simulink library "dspsnks2"  (Simulink 3.00)
undefined symbols (not defined in the file or in its folder): get, hot
libraries: dspspect2 x2, dspmtrx2 x2, dspbuff2 x1, dspsnks2 x1
settings Model: Creator=don  LastModifiedBy=don

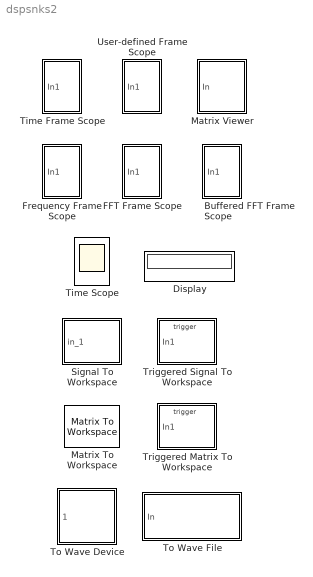
== system dspsnks2 ==
  Buffered FFT Frame Scope : Subsystem  mask(Buffered FFT Frame Scope){FFTlength=128, BufferSize=128, Overlap=64, Domain=Frequency, XLabel=Samples, XUnits=Hertz, XRange=[0...Fs/2], XIncr=-1, YLabel=Magnitude, dB, YUnits=dB, HorizSpan=1, NChans=1, AxisParams=off, YMin=-10, YMax=10, FigPos=get(0,'defaultfigureposition'), AxisGrid=on, AxisZoom=on, FrameNumber=off, AxisLegend=off, Memory=off, LineParams=off, LineDisables=, LineColors=, LineStyles=, LineMarkers=}
      mask prompts: FFTlength "FFT length (-1 to inherit input width):"; BufferSize "Buffer size:"; Overlap "Buffer overlap:"; Domain "Input domain:"; XLabel "X-axis title:"; XUnits "Frequency units:"; XRange "Frequency range:"; XIncr "Sample time of original time series (-1 if not zero-padded):"; YLabel "Y-axis title:"; YUnits "Amplitude scaling:"; HorizSpan "Time display span (number of frames):"; NChans "Number of input channels:"; AxisParams "Axis properties ..."; YMin "Minimum Y-limit:"; YMax "Maximum Y-limit:"; FigPos "Figure position:"; AxisGrid "Axis grid"; AxisZoom "Axis zoom"; FrameNumber "Frame number"; AxisLegend "Axis legend"; LineParams "Line properties ..."; LineDisables "Line visibility:"; LineColors "Line colors:"; LineStyles "Line styles:"; LineMarkers "Line markers:"
      mask help: Buffer a non-frame based input, then compute and display the magnitude-squared FFT of each each frame of input data.
      mask init:
      | [x,y,str] = dspblkbfftscope('icon');
      | s = dspblkbfftscope('init',FFTlength,BufferSize,Overlap,Domain, XLabel, XUnits, XRange, XIncr, ...
      | YLabel, YUnits,  HorizSpan, NChans, ...
      | AxisParams, YMin,YMax,FigPos, ...
      | AxisGrid, AxisZoom, FrameNumber, AxisLegend, Memory, ...
      | LineParams, LineDisables, LineColors, LineStyles, LineMarkers);
      settings: CopyFcn=sdspfscope([],[],[],'BlockCopy');  DeleteFcn=sdspfscope([],[],[],'BlockDelete');  NameChangeFcn=sdspfscope([],[],[],'NameChange');
      mask Help: web(dspbhelp);
      mask StyleString: edit,edit,edit,popup(Time|Frequency|User-defined),edit,popup(Hertz|rad/sec),popup([0...Fs/2]|[-Fs/2...Fs/2]|[0...Fs]),edit,edit,popup(Magnitude|dB),edit,edit,checkbox,edit,edit,edit,checkbox,checkbox,checkbox,checkbox,checkbox,checkbox,edit,edit,edit,edit
      mask CallbackString: |||dspblkbfftscope('dynamic','Domain');|||||||||dspblkbfftscope('dynamic','AxisParams');|||||||||dspblkbfftscope('dynamic','LineParams');||||
      mask Display: plot(x,y); text(14,20,str);
  Display : Display
      settings: Format=short
  FFT Frame Scope : Subsystem  mask(FFT Frame Scope){FFTlength=128, Domain=Frequency, XLabel=Samples, XUnits=Hertz, XRange=[0...Fs/2], XIncr=-1, YLabel=Magnitude, dB, YUnits=dB, HorizSpan=1, NChans=1, AxisParams=off, YMin=-10, YMax=10, FigPos=get(0,'defaultfigureposition'), AxisGrid=on, AxisZoom=on, FrameNumber=off, AxisLegend=off, Memory=off, LineParams=off, LineDisables=, LineColors=, LineStyles=, LineMarkers=}
      mask prompts: FFTlength "FFT length (-1 to inherit input width):"; Domain "Input domain:"; XLabel "X-axis title:"; XUnits "Frequency units:"; XRange "Frequency range:"; XIncr "Sample time of original time series (-1 if not zero-padded):"; YLabel "Y-axis title:"; YUnits "Amplitude scaling:"; HorizSpan "Time display span (number of frames):"; NChans "Number of input channels:"; AxisParams "Axis properties ..."; YMin "Minimum Y-limit:"; YMax "Maximum Y-limit:"; FigPos "Figure position:"; AxisGrid "Axis grid"; AxisZoom "Axis zoom"; FrameNumber "Frame number"; AxisLegend "Axis legend"; LineParams "Line properties ..."; LineDisables "Line visibilities:"; LineColors "Line colors:"; LineStyles "Line styles:"; LineMarkers "Line markers:"
      mask help: Compute and display the magnitude-squared FFT of a frame of time-domain input data.
      mask init:
      | [x,y,str] = dspblkfftscope('icon');
      | s = dspblkfftscope('init',FFTlength,Domain, XLabel, XUnits, XRange, XIncr, ...
      | YLabel, YUnits,  HorizSpan, NChans, ...
      | AxisParams, YMin,YMax,FigPos, ...
      | AxisGrid, AxisZoom, FrameNumber, AxisLegend, Memory, ...
      | LineParams, LineDisables, LineColors, LineStyles, LineMarkers);
      settings: CopyFcn=sdspfscope([],[],[],'BlockCopy');  DeleteFcn=sdspfscope([],[],[],'BlockDelete');  NameChangeFcn=sdspfscope([],[],[],'NameChange');
      mask Help: web(dspbhelp);
      mask StyleString: edit,popup(Time|Frequency|User-defined),edit,popup(Hertz|rad/sec),popup([0...Fs/2]|[-Fs/2...Fs/2]|[0...Fs]),edit,edit,popup(Magnitude|dB),edit,edit,checkbox,edit,edit,edit,checkbox,checkbox,checkbox,checkbox,checkbox,checkbox,edit,edit,edit,edit
      mask CallbackString: |dspblkfftscope('dynamic','Domain');|||||||||dspblkfftscope('dynamic','AxisParams');|||||||||dspblkfftscope('dynamic','LineParams');||||
      mask Display: plot(x,y); text(14,20,str);
  Frequency Frame Scope : Subsystem  mask(Frequency Frame Scope){Domain=Frequency, XLabel=Samples, XUnits=Hertz, XRange=[0...Fs/2], XIncr=-1, YLabel=Magnitude, dB, YUnits=dB, HorizSpan=1, NChans=1, AxisParams=off, YMin=-10, YMax=10, FigPos=get(0,'defaultfigureposition'), AxisGrid=on, AxisZoom=on, FrameNumber=off, AxisLegend=off, Memory=off, LineParams=off, LineDisables=, LineColors=, LineStyles=, LineMarkers=}
      mask prompts: Domain "Input domain:"; XLabel "X-axis title:"; XUnits "Frequency units:"; XRange "Frequency range:"; XIncr "Sample time of original time series (-1 if not zero-padded):"; YLabel "Y-axis title:"; YUnits "Amplitude scaling:"; HorizSpan "Time display span (number of frames):"; NChans "Number of input channels:"; AxisParams "Axis properties ..."; YMin "Minimum Y-limit:"; YMax "Maximum Y-limit:"; FigPos "Figure position:"; AxisGrid "Axis grid"; AxisZoom "Axis zoom"; FrameNumber "Frame number"; AxisLegend "Axis legend"; LineParams "Line properties ..."; LineDisables "Line visibilities:"; LineColors "Line colors:"; LineStyles "Line styles:"; LineMarkers "Line markers:"
      mask help: Display one or more frequency domain data sets. Data should come from an FFT block, or from frequency-domain sources with equivalent data organization.
      mask init:
      | [x,y,str] = dspblkfscope('icon');
      | s = dspblkfscope('init',Domain, XLabel, XUnits, XRange, XIncr, ...
      | YLabel, YUnits,  HorizSpan, NChans, ...
      | AxisParams, YMin,YMax,FigPos, ...
      | AxisGrid, AxisZoom, FrameNumber, AxisLegend, Memory, ...
      | LineParams, LineDisables, LineColors, LineStyles, LineMarkers);
      settings: CopyFcn=sdspfscope([],[],[],'BlockCopy');  DeleteFcn=sdspfscope([],[],[],'BlockDelete');  NameChangeFcn=sdspfscope([],[],[],'NameChange');
      mask Help: web(dspbhelp);
      mask StyleString: popup(Time|Frequency|User-defined),edit,popup(Hertz|rad/sec),popup([0...Fs/2]|[-Fs/2...Fs/2]|[0...Fs]),edit,edit,popup(Magnitude|dB),edit,edit,checkbox,edit,edit,edit,checkbox,checkbox,checkbox,checkbox,checkbox,checkbox,edit,edit,edit,edit
      mask CallbackString: dspblkfscope('dynamic','Domain');|||||||||dspblkfscope('dynamic','AxisParams');|||||||||dspblkfscope('dynamic','LineParams');||||
      mask Display: plot(x,y); text(14,20,str);
  Matrix To Workspace : dspmtrx2/Matrix To Workspace  matname=yout  maxrows=1000  deci=1  matsiz=[3 3]
  Matrix Viewer : Subsystem  mask(Matrix Viewer){ImageParams=off, CMap=hot(256), YMin=-1.0, YMax=1.0, NumCols=10, AxisColorbar=on, AxisParams=off, AxisOrigin=Upper left corner, XLabel=X-axis, YLabel=Y-axis, ZLabel=Z-axis, FigPos=get(0,'defaultfigureposition'), AxisZoom=off}
      mask prompts: ImageParams "Image properties ..."; CMap "Colormap matrix:"; YMin "Minimum input value:"; YMax "Maximum input value:"; NumCols "Number of columns:"; AxisColorbar "Display colorbar"; AxisParams "Axis properties ..."; AxisOrigin "Axis origin:"; XLabel "X-axis title:"; YLabel "Y-axis title:"; ZLabel "Colorbar title:"; FigPos "Figure position:"; AxisZoom "Axis zoom"
      mask help: Display a matrix as an image, scaling the colormap to the specified input data range. Colormap must be an Nx3 matrix of RGB values. Type "help graph3d" at the MATLAB prompt for a list of predefined colormaps.
      mask init:
      | s = dspblkmview('init', ...
      |        ImageParams, CMap, YMin, YMax, NumCols, AxisColorbar,  ...
      |        AxisParams,  AxisOrigin, XLabel,  YLabel,  ZLabel, FigPos, AxisZoom);
      settings: CopyFcn=sdspmview([],[],[],'BlockCopy');  DeleteFcn=sdspmview([],[],[],'BlockDelete');  NameChangeFcn=sdspmview([],[],[],'NameChange');
      mask Help: web(dspbhelp);
      mask StyleString: checkbox,edit,edit,edit,edit,checkbox,checkbox,popup(Upper left corner|Lower left corner),edit,edit,edit,edit,checkbox
      mask CallbackString: dspblkmview('dynamic','ImageParams');||||||dspblkmview('dynamic','AxisParams');||||||
      mask Display: disp('Matrix\nViewer');
  Signal To Workspace : Subsystem  mask(Signal To Workspace){VariableName=yout, Buffer=1000, Decimation=1, FrameBased=off, NumChans=1}
      mask prompts: VariableName "Variable name:"; Buffer "Maximum number of inputs to record:"; FrameBased "Frame-based"; NumChans "Number of channels:"
      mask help: Write input to specified matrix in the workspace. The matrix has one column per input element and one row per time step. For frame-based operation, note that each simulation step may represent multiple time steps. Data is not available until the simulation is stopped or paused.
      mask Help: web(dspbhelp);
      mask CallbackString: |||dspblkstw|
      mask Display: disp(VariableName)
  Time Frame Scope : Subsystem  mask(Time Frame Scope){Domain=Time, XLabel=Samples, XUnits=Hertz, XRange=[0...Fs/2], XIncr=-1, YLabel=Amplitude, YUnits=dB, HorizSpan=1, NChans=1, AxisParams=off, YMin=-10, YMax=10, FigPos=get(0,'defaultfigureposition'), AxisGrid=on, AxisZoom=on, FrameNumber=off, AxisLegend=off, Memory=off, LineParams=off, LineDisables=, LineColors=, LineStyles=, LineMarkers=}
      mask prompts: Domain "Input domain:"; XLabel "X-axis title:"; XUnits "Frequency units:"; XRange "Frequency range:"; XIncr "Sample time of original time series (-1 if not zero-padded):"; YLabel "Y-axis title:"; YUnits "Amplitude scaling:"; HorizSpan "Time display span (number of frames):"; NChans "Number of input channels:"; AxisParams "Axis properties ..."; YMin "Minimum Y-limit:"; YMax "Maximum Y-limit:"; FigPos "Figure position:"; AxisGrid "Axis grid"; AxisZoom "Axis zoom"; FrameNumber "Frame number"; AxisLegend "Axis legend"; LineParams "Line properties ..."; LineDisables "Line visibilities:"; LineColors "Line colors:"; LineStyles "Line styles:"; LineMarkers "Line markers:"
      mask help: Display a vector or matrix of data frames. Data should come from frame-based, time-domain sources.
      mask init: same as dspsnks2/Frequency Frame Scope
      settings: CopyFcn=sdspfscope([],[],[],'BlockCopy');  DeleteFcn=sdspfscope([],[],[],'BlockDelete');  NameChangeFcn=sdspfscope([],[],[],'NameChange');
      mask Help: web(dspbhelp);
      mask StyleString: popup(Time|Frequency|User-defined),edit,popup(Hertz|rad/sec),popup([0...Fs/2]|[-Fs/2...Fs/2]|[0...Fs]),edit,edit,popup(Magnitude|dB),edit,edit,checkbox,edit,edit,edit,checkbox,checkbox,checkbox,checkbox,checkbox,checkbox,edit,edit,edit,edit
      mask CallbackString: dspblkfscope('dynamic','Domain');|||||||||dspblkfscope('dynamic','AxisParams');|||||||||dspblkfscope('dynamic','LineParams');||||
      mask Display: plot(x,y); text(14,20,str);
  Time Scope : Scope
      settings: TimeRange=auto  YMin=-5  YMax=5  SaveToWorkspace=off  SaveName=ScopeData  DataFormat=Structure
  To Wave Device : Subsystem  mask(To Wave Device){sampleWidthLit=16, stereo=off, bufDuration=2, initDelay=0.1, useDefaultDevice=on, userDeviceID=1}
      mask prompts: sampleWidthLit "Sample width (bits):"; bufDuration "Queue duration (seconds):"; initDelay "Initial output delay (seconds):"; useDefaultDevice "Use default audio device"; userDeviceID "Audio device ID: (1=1st device, 2=2nd device, ...)"
      mask help: Writes audio data samples to a standard Windows audio device in real time. If audio glitches occur, increase Initial output delay (for glitches at startup) or Queue duration. Only for Win95/98/NT.
      mask init:
      | [x,y,x1,y1,x2,y2] = dspblkwao('icon');
      | [bits_per_sample, numChannels, deviceID] = dspblkwao('init',userDeviceID);
      mask Help: web(dspbhelp);
      mask StyleString: popup(8|16),checkbox,edit,edit,checkbox,edit
      mask CallbackString: ||||dspblkwao;|
      mask Display:
      | patch(x1,y1,[1 1 1]*.5);
      | patch(x2,y2);
      | plot(x,y); plot(x1,y1)
  To Wave File : Subsystem  mask(To Wave File){filename=audio, sampleWidth=16, stereo=off}
      mask prompts: filename "File name:"; sampleWidth "Sample width (bits):"
      mask help: Writes audio data samples to a standard Windows PCM format ".WAV" audio file. Only for Win95/98/NT.
      mask init:
      | col_major=1;
      | numChannels=1+stereo;
      | bits_per_sample=str2num(sampleWidth);
      | if ~strcmp(lower(filename(end-3:end)),'.wav'), filename=strcat(filename,'.wav');end
      mask Help: web(dspbhelp);
      mask StyleString: edit,popup(8|16),checkbox
      mask Display: disp(filename)
  Triggered Matrix To Workspace : Subsystem  mask(Triggered Matrix To Workspace){TriggerType=Rising edge, matname=yout, maxrows=1000, deci=1, matsiz=[3 3]}
      mask prompts: TriggerType "Trigger type:"; matname "Variable name:"; maxrows "Maximum number of matrices:"; deci "Decimation:"; matsiz "Matrix size:"
      mask help: Write a matrix signal into the workspace, storing the resulting time-sequence as a 3-D array with time running along the third dimension. Data is not available until the simulation is stopped or paused.
      mask init:
      | child=['Matrix' sprintf('\n') 'To Workspace'];
      | switch TriggerType
      | case 1, s='rising';
      | case 2, s='falling';
      | case 3, s='either';
      | end
      | if ~strcmp(get_param([gcb '/Trigger'],'TriggerType'),s)
      |      set_param([gcb '/Trigger'],'TriggerType',s);
      | end;
      | if ~strcmp(get_param([gcb '/' child],'matname'),matname)
      |      set_param([gcb '/' child],'matname',matname);
      | end;
      mask Help: web(dspbhelp);
      mask StyleString: popup(Rising edge|Falling edge|Either edge),edit,edit,edit,edit
      mask Display: disp(matname);
  Triggered Signal To Workspace : Subsystem  mask(Triggered Signal To Workspace){TriggerType=Rising edge, VariableName=yout, Buffer=1000, Decimation=1, FrameBased=off, NumChans=1}
      mask prompts: TriggerType "Trigger type:"; VariableName "Variable name:"; Buffer "Maximum number of rows:"; FrameBased "Frame-based"; NumChans "Number of channels:"
      mask help: Write input to specified matrix in the workspace when trigger is received. The matrix has one column per input element and one row per time step. For frame-based operation, note that each simulation step may represent multiple time steps. Data is not available until the simulation is stopped or paused.
      mask init:
      | dspblktstw('init',TriggerType, VariableName, Buffer, Decimation, FrameBased, NumChans);
      mask Help: web(dspbhelp);
      mask StyleString: popup(Rising edge|Falling edge|Either edge),edit,edit,edit,checkbox,edit
      mask CallbackString: ||||dspblktstw('dynamic');|
      mask Display: disp(VariableName);
  User-defined Frame Scope : Subsystem  mask(User-defined Frame Scope){Domain=User-defined, XLabel=Samples, XUnits=Hertz, XRange=[0...Fs/2], XIncr=-1, YLabel=Magnitude, dB, YUnits=dB, HorizSpan=1, NChans=1, AxisParams=off, YMin=-10, YMax=10, FigPos=get(0,'defaultfigureposition'), AxisGrid=on, AxisZoom=on, FrameNumber=off, AxisLegend=off, Memory=off, LineParams=off, LineDisables=, LineColors=, LineStyles=, LineMarkers=}
      mask prompts: Domain "Input domain:"; XLabel "X-axis title:"; XUnits "Frequency units:"; XRange "Frequency range:"; XIncr "Increment per sample in input frame:"; YLabel "Y-axis title:"; YUnits "Amplitude scaling:"; HorizSpan "Horizontal display span (number of frames):"; NChans "Number of input channels:"; AxisParams "Axis properties ..."; YMin "Minimum Y-limit:"; YMax "Maximum Y-limit:"; FigPos "Figure position:"; AxisGrid "Axis grid"; AxisZoom "Axis zoom"; FrameNumber "Frame number"; AxisLegend "Axis legend"; LineParams "Line properties ..."; LineDisables "Line visibilities:"; LineColors "Line colors:"; LineStyles "Line styles:"; LineMarkers "Line markers:"
      mask help: Display a vector or matrix of data frames. Data should be from frame-based, user-defined data sources.
      mask init: same as dspsnks2/Frequency Frame Scope
      settings: CopyFcn=sdspfscope([],[],[],'BlockCopy');  DeleteFcn=sdspfscope([],[],[],'BlockDelete');  NameChangeFcn=sdspfscope([],[],[],'NameChange');
      mask Help: web(dspbhelp);
      mask StyleString: popup(Time|Frequency|User-defined),edit,popup(Hertz|rad/sec),popup([0...Fs/2]|[-Fs/2...Fs/2]|[0...Fs]),edit,edit,popup(Magnitude|dB),edit,edit,checkbox,edit,edit,edit,checkbox,checkbox,checkbox,checkbox,checkbox,checkbox,edit,edit,edit,edit
      mask CallbackString: dspblkfscope('dynamic','Domain');|||||||||dspblkfscope('dynamic','AxisParams');|||||||||dspblkfscope('dynamic','LineParams');||||
      mask Display: plot(x,y); text(14,20,str);

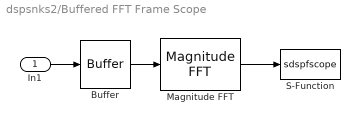
== system dspsnks2/Buffered FFT Frame Scope ==
  In1 : Inport  Port=1  PortWidth=-1  SampleTime=-1  DataType=auto
      settings: SignalType=auto
  Buffer : dspbuff2/Buffer  N=BufferSize  V=Overlap  ic=0
  Magnitude FFT : dspspect2/Magnitude FFT  fftsize=FFTlength  NChans=NChans
  S-Function : S-Function  FunctionName=sdspfscope  Parameters=s  PortCounts=[]  SFunctionModules=''
  wires:
  Magnitude FFT/1 -> S-Function/1
  In1/1 -> Buffer/1
  Buffer/1 -> Magnitude FFT/1

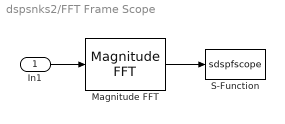
== system dspsnks2/FFT Frame Scope ==
  In1 : Inport  Port=1  PortWidth=-1  SampleTime=-1  DataType=auto
      settings: SignalType=auto
  Magnitude FFT : dspspect2/Magnitude FFT  fftsize=FFTlength  NChans=NChans
  S-Function : S-Function  FunctionName=sdspfscope  Parameters=s  PortCounts=[]  SFunctionModules=''
  wires:
  In1/1 -> Magnitude FFT/1
  Magnitude FFT/1 -> S-Function/1

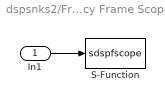
== system dspsnks2/Frequency Frame Scope ==
  In1 : Inport  Port=1  PortWidth=-1  SampleTime=-1  DataType=auto
      settings: SignalType=auto
  S-Function : S-Function  FunctionName=sdspfscope  Parameters=s  PortCounts=[]  SFunctionModules=''
  wires:
  In1/1 -> S-Function/1

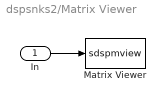
== system dspsnks2/Matrix Viewer ==
  In : Inport  Port=1  PortWidth=-1  SampleTime=-1  DataType=auto
      settings: SignalType=auto
  Matrix Viewer : S-Function  FunctionName=sdspmview  Parameters=s  PortCounts=[]  SFunctionModules=''
  wires:
  In/1 -> Matrix Viewer/1

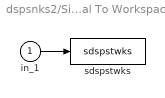
== system dspsnks2/Signal To Workspace ==
  in_1 : Inport  Port=1  PortWidth=-1  SampleTime=-1  DataType=auto
      settings: SignalType=auto
  sdspstwks : S-Function  FunctionName=sdspstwks  Parameters=VariableName,Buffer,Decimation,FrameBased,NumChans  PortCounts=[]  SFunctionModules=''
  wires:
  in_1/1 -> sdspstwks/1

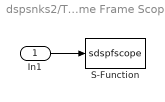
== system dspsnks2/Time Frame Scope ==
  In1 : Inport  Port=1  PortWidth=-1  SampleTime=-1  DataType=auto
      settings: SignalType=auto
  S-Function : S-Function  FunctionName=sdspfscope  Parameters=s  PortCounts=[]  SFunctionModules=''
  wires:
  In1/1 -> S-Function/1

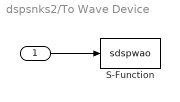
== system dspsnks2/To Wave Device ==
  " " : Inport  Port=1  PortWidth=-1  SampleTime=-1  DataType=auto
      settings: SignalType=auto
  S-Function : S-Function  FunctionName=sdspwao  Parameters=numChannels, bits_per_sample, bufDuration, initDelay, deviceID  PortCounts=[]  SFunctionModules=winmm.lib
  wires:
  " "/1 -> S-Function/1

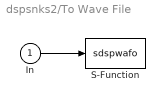
== system dspsnks2/To Wave File ==
  In : Inport  Port=1  PortWidth=-1  SampleTime=-1  DataType=auto
      settings: SignalType=auto
  S-Function : S-Function  FunctionName=sdspwafo  Parameters=filename, bits_per_sample, numChannels  PortCounts=[]  SFunctionModules=winmm.lib
  wires:
  In/1 -> S-Function/1

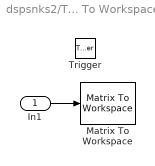
== system dspsnks2/Triggered Matrix To Workspace ==
  In1 : Inport  Port=1  PortWidth=-1  SampleTime=-1  DataType=auto
      settings: SignalType=auto
  Trigger : TriggerPort  TriggerType=rising  OutputDataType=auto
  Matrix To Workspace : dspmtrx2/Matrix To Workspace  matname=yout  maxrows=maxrows  deci=deci  matsiz=matsiz
  wires:
  In1/1 -> Matrix To Workspace/1

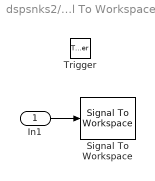
== system dspsnks2/Triggered Signal To Workspace ==
  In1 : Inport  Port=1  PortWidth=-1  SampleTime=-1  DataType=auto
      settings: SignalType=auto
  Trigger : TriggerPort  TriggerType=rising  OutputDataType=auto
  Signal To Workspace : dspsnks2/Signal To Workspace  VariableName=yout  Buffer=Buffer  FrameBased=off  NumChans=NumChans
      settings: Decimation=Decimation
  wires:
  In1/1 -> Signal To Workspace/1

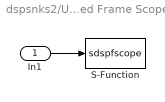
== system dspsnks2/User-defined Frame Scope ==
  In1 : Inport  Port=1  PortWidth=-1  SampleTime=-1  DataType=auto
      settings: SignalType=auto
  S-Function : S-Function  FunctionName=sdspfscope  Parameters=s  PortCounts=[]  SFunctionModules=''
  wires:
  In1/1 -> S-Function/1
